simulink model "VSC_GFo_Fixed_Frequency_variable"  (R2016a)
settings: Solver=ode23tb  SolverMode=SingleTasking  StartTime=0.0  StopTime=2  FixedStep=Time_Step  MaxStep=1e-5  RelTol=1e-3
PreLoadFcn:
  | VSC_GFo_Init;
InitFcn:
  | VSC_GFo_Init;
values from neighbouring files (symbols this model uses):
  fb = fn    (= 50)    [VSC_GFo_Init.m]
  fn = 50    [VSC_GFo_Init.m]
  GRD00_Lg = GRD00_Xg/wb    (= 0.0254647908947)    [VSC_GFo_Init.m]
  GRD00_Rg = GRD00_Rg_pu*GRD00_Zb    (= 0.8)    [VSC_GFo_Init.m]
  Time_Step = 50e-6    (= 5e-05)    [VSC_GFo_Init.m]
  VSC01_Delta_P_Time_Step = 0.2    [VSC_GFo_Init.m]
  VSC01_Delta_P_Value = 0.2    [VSC_GFo_Init.m]
  VSC01_Udc_n = 640 * 1e3    (= 640000)    [VSC_GFo_Init.m]
undefined symbols (not defined in the file or in its folder): DiscIntNeverNeededParam, VSC01_id0
undefined symbols (not defined in the file): GRD00_H, GRD00_R, GRD00_TD, GRD00_TN, GRD00_Ub, VSC01_DX_DR, VSC01_I_thresh_pu, VSC01_Kp_Rvi_pu, VSC01_Lt_pu, VSC01_mp1, VSC01_mp2, VSC01_mp3, VSC01_Pn, VSC01_R, VSC01_Rt_pu, VSC01_Rv, VSC01_Sn, VSC01_T1, VSC01_T2, VSC01_Un1, VSC01_Un2, VSC01_W_LF, VSC01_wc1, VSC01_wc2, VSC01_wc3
libraries: powerlib x20, simulink x3, powerlib_meascontrol x1
(part 1 of 2)
settings Model: Creator=Frederic_Colas  LastModifiedBy=Frederic_Colas
settings DebuggingCC: UnconnectedInputMsg=none  UnconnectedOutputMsg=none  UnconnectedLineMsg=none  SFUnexpectedBacktrackingDiag=error  SFNoUnconditionalDefaultTransitionDiag=error
settings HardwareCC: ProdWordSize=32  ProdHWDeviceType=Specified
settings GRTTargetCC: TargetLangStandard=C99 (ISO)  GeneratePreprocessorConditionals=Use local settings
settings ConfigComp: CovMetricSettings=dwe  CovHtmlReporting=off  CovSaveCumulativeToWorkspaceVar=off  CovSaveSingleToWorkspaceVar=off  CovExternalEMLEnable=on
settings SimscapeCC: SimscapeNormalizeSystem=off

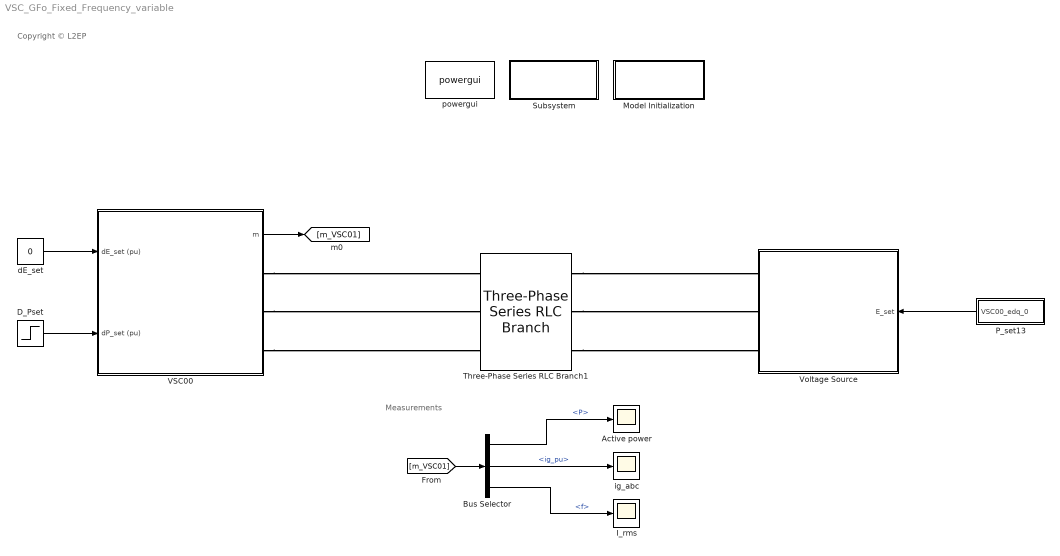
== system VSC_GFo_Fixed_Frequency_variable ==
  note: Copyright © L2EP
  note: Measurements
  Active power : Scope
  Bus Selector : BusSelector  OutputSignals=Control.P,ig_pu,Control.f
  D_Pset : Step  Time=VSC01_Delta_P_Time_Step  After=VSC01_Delta_P_Value  SampleTime=0
  I_rms : Scope
  Model Initialization : Subsystem  mask(Model Functions){InitFcnX=VSC_GFo_Init;, prel=on, posl=off, inif=on, strf=off}
      mask prompts: InitFcnX "Initialisation"; prel "Preload Function"; posl "PostLoad Function"; inif "InitFcn"; strf "StartFcn"
      mask init:
      | currentBlock = gcb;
      | root = bdroot(currentBlock);
      | 
      | if ~strcmp(get_param(root,'BlockDiagramType'),'library')
      |     if prel==1
      |         set_param(root, 'PreLoadFcn', InitFcnX);
      |     else
      |         set_param(root, 'PreLoadFcn', '');
      |     end
      |     if inif==1
      |         set_param(root, 'InitFcn', InitFcnX);
      |     else
      |         set_param(root, 'InitFcn', '');
      |     end
      |     if strf==1
      |         set_param(root, 'StartFcn', InitFcnX);
      |     else
      |         set_param(root, 'StartFcn', '');
      |     end
      |     if posl==1
      |         set_param(root, 'PostLoadFcn', InitFcnX);
      |     else
      |         set_param(root, 'PostLoadFcn', '');
      |     end
      | end
      | 
      | pos = get_param(currentBlock, 'Position');
      | width = pos(3) - pos(1); height = pos(4) - pos(2);
      | txt = [ upper(root) '\n' '- InitFcn. . . . . '  get_param(root, 'InitFcn') ];
      settings: CopyFcn=set_param(gcb,'LinkStatus','none')
      mask Display:
      | %text(5, height*0.5, txt, 'horizontalAlignment', 'left', 'verticalAlignment', 'middle') ;
      | color('blue'),disp('Initialization Function\nParameters')
  P_set13 : Subsystem
  Subsystem : Subsystem
      settings: OpenFcn=LoadFlow_VSC_v2
      mask Display: color('blue'),disp('Update Loadflow')
  Three-Phase Series RLC Branch1 : powerlib/Elements/Three-Phase Series RLC Branch  LConnTagsString=A|B|C  RConnTagsString=A|B|C  BranchType=RL  Resistance=GRD00_Rg  Inductance=GRD00_Lg  Capacitance=1e-6  Measurements=None
  VSC00 : Subsystem  mask(VSC){fb=fb, Sn=VSC01_Sn, Pn=VSC01_Pn, Vdcn=VSC01_Udc_n, Un1=VSC01_Un1, Un2=VSC01_Un2, Rt_pu=VSC01_Rt_pu, Lt_pu=VSC01_Lt_pu, Lm_pu=500, Rm_pu=500, Tr_PLL=100e-3, Val_Freq_Support=on, R_percent=VSC01_R, Rv=VSC01_Rv, W_TVR=VSC01_W_LF, I_thresh_pu=VSC01_I_thresh_pu, DX_DR=VSC01_DX_DR, Kp_Rvi_pu=VSC01_Kp_Rvi_pu, gainpopup=1, wc1=VSC01_wc1, mp1=VSC01_mp1, wc2=VSC01_wc2, mp2=VSC01_mp2, wc3=VSC01_wc3, mp3=VSC01_mp3, T1=VSC01_T1, T2=VSC01_T2, LFpopup=PQ, P0=0.5, Q0=5.2102e-06, V0=1, Theta0=1.4294}
      mask prompts: fb "Nominal Frequency (Hz)"; Sn "Nominal Apparent Power (VA)"; Pn "Nominal Power (W)"; Vdcn "Nominal DC Voltage (V)"; Un1 "VSC side Nominal Ph-Ph Voltage (V)"; Un2 "Grid side Nominal Ph-Ph Voltage (V)"; Rt_pu "R (pu)"; Lt_pu "L (pu)"; Lm_pu "Rm (pu)"; Rm_pu "Lm (pu)"; Tr_PLL "Time response (s)"; Val_Freq_Support "Frequency Support"; R_percent "Droop Gain (%)"; Rv "Damping Resistance (Rv)"; W_TVR "Dr filter"; I_thresh_pu "Current Threshold (pu)"; Kp_Rvi_pu "Kp_Rvi"; gainpopup "Strategy"; wc1 "wc"; mp1 "mp"; wc2 "wc"; mp2 "mp"; wc3 "wc"; mp3 "mp"; P0 "Initial Active Power (pu)"; Q0 "Initial Reactive Power (pu)"; V0 "Initial Voltage (pu)"; Theta0 "Initial Angle (°)"
      mask init:
      | % Update Name of LF bus for internal purpose
      |     NameStr = [get_param(gcb,'Name')];% '_LF'];
      |     set_param([gcb '/Load Flow Bus'],'ID',NameStr);
      |     %disp(NameStr);
      |     
      | % Increase size of Mask dialog box
      |    % pause(0.1);
      |     
      |     
      | % Base values
      |     %Un = Un1;
      |     Pb = Pn;
      |     cos_phi_n = Pn/Sn;
      |     Sb = Pb/cos_phi_n;
      |     %Ub = Un;
      |     Vn = Un1/sqrt(3);
      |     Vb = Vn;
      |     %Ib = Sb / Ub;
      |     Ib = Sb / (3*Vb);
      |     wb = 2*pi*fb;
      |   
      | % PLL derivation of the parameters
      |     wn_PLL=5/Tr_PLL;
      |     zeta_PLL = 1;
      |     Kp_PLL_pu = 2*zeta_PLL*wn_PLL/wb;
      |     Ki_PLL_pu = wn_PLL^2/wb;
      |     
      | % Set the chosen strategy
      |     Chosen_Strategy = gainpopup;
      |     
      | % Set the frequency droop gain
      |     R = R_percent;
      | 
      | % Compute Initial Voltage of VSC 
      | %   from steady-state output transformer model and Loadflow result
      |     if (LFpopup == 'PQ')
      |         V0 = 1;
      |     end
      |         
      |     R1_pu = Rt_pu/2;
      |     L1_pu = Lt_pu/2;
      |     R2_pu = Rt_pu/2;
      |     L2_pu = Lt_pu/2;
      |     X1_pu = L1_pu;
      |     X2_pu = L2_pu;
      |     Xm_pu = Lm_pu;
      |     
      |     Zm_pu = 1/(1/Rm_pu+1/(1i*Xm_pu));
      | 
      |     S0=P0+1i*Q0;
      |     I2 = conj(S0)/(V0);
      | 
      |     Vm = (R2_pu+1i*X2_pu)*I2 + V0;
      |     Im = Vm/Zm_pu;
      | 
      |     I1 = I2 + Im;
      |     V1 = (R1_pu+1i*X1_pu) * I1 + Vm;
      | 
      |     Vvsc0 = abs(V1);
      |    % disp(Vvsc0*1000)
      |     Theta_vsc0 = angle(V1) * 180/pi+Theta0;
      |     
      |     %vd0=Vvsc0*cos(Theta0*2*pi/180);
      |     %vq0=Vvsc0*sin(Theta0*2*pi/180); 
      |  
      |     %Va0 = Vvsc0*sqrt(2)*Ub/sqrt(3)*sin(Theta_vsc0*pi/180);
      |     %Vb0 = Vvsc0*sqrt(2)*Ub/sqrt(3)*sin(Theta_vsc0*pi/180-2*pi/3);
      |     %Vc0 = Vvsc0*sqrt(2)*Ub/sqrt(3)*sin(Theta_vsc0*pi/180+2*pi/3);
      |     
      |     Va0 = Vvsc0*sqrt(2)*Vb*sin(Theta_vsc0*pi/180);
      |     Vb0 = Vvsc0*sqrt(2)*Vb*sin(Theta_vsc0*pi/180-2*pi/3);
      |     Vc0 = Vvsc0*sqrt(2)*Vb*sin(Theta_vsc0*pi/180+2*pi/3);
      |     
      | % Generate string to display LF results on Mask
      |     %str_tmp = fprintf("Vvsc0 = %d, Theta_vsc0 = %d°",Vvsc0,Theta_vsc0);
      |     mo = get_param(gcb,'MaskObject');
      |     mo.getDialogControl('LF_vsc_str').Prompt = ['V0 = ', num2str(Vvsc0),' pu, Angle = ', num2str(Theta_vsc0),'°'];
      |     mo.getDialogControl('LF_pcc_str').Prompt = ['V0 = ', num2str(V0),' pu, Angle = ', num2str(Theta0),'°'];
      |     mo.getDialogControl('LF_pcc_Power_str').Prompt = ['P0 = ', num2str(P0),' pu, Q0 = ', num2str(Q0),' pu'];
      |     %set_param([gcb],'LF_str',str_tmp);
      |  %GRD00_Theta0 = Theta0;
      |  %P0 = 200e6;
      |  %Q0 = 0;
      |  % Initial current values of VSC (dq pu) 
      |  %id0 =(P0*vd0+Q0*vq0)/(vd0^2+vq0^2) * 1/Ib; %
      |  %iq0 =(P0*vq0-Q0*vd0)/(vd0^2+vq0^2) * 1/Ib; %Initial current in the connexion inductance
      settings: OpenFcn=|
      | NameStr = get_param(gcb,'Name');
      | open_system(gcbh, 'Mask');
      | 
      | h2AllOpenDlgs = DAStudio.ToolRoot.getOpenDialogs;
      | 
      | for i=1:length(h2AllOpenDlgs)
      |     try
      |          %disp(h2AllOpenDlgs(i).getSource.getBlock.Name);
      |         Dialog_block_name = h2AllOpenDlgs(i).getSource.getBlock.Name;
      |          %strcmp(Dialog_block_name, NameStr),
      |         if (strcmp(h2AllOpenDlgs(i).getSource.getBlock.Name, NameStr))
      |             iPos = h2AllOpenDlgs(i).position;
      |             h2AllOpenDlgs(i).position = [iPos(1)   iPos(2)   iPos(3)*1.4   iPos(4)];
      |         end
      |     end
      | end
      mask TypeOptions gainpopup: 1 | 2 | 3
      mask Callback gainpopup:
      | % Get the mask parameter values. This is a cell
      | %   array of character vectors.
      | maskStr = get_param(gcb,'gainpopup');
      | p=Simulink.Mask.get(gcb);
      | 
      | % The pop-up menu is the first mask parameter.
      | %   Check the value selected in the pop-up
      | if strcmp(maskStr,'1'),
      | 
      |     % Set the visibility of both parameters on when
      |     %   User-defined is selected in the pop-up.
      |     p.getDialogControl('Param_Strat_1').Visible='on';
      |     p.getDialogControl('Param_Strat_2').Visible='off';
      |     p.getDialogControl('Param_Strat_3').Visible='off';
      | 
      | elseif strcmp(maskStr,'2'),
      | 
      |     % Set the visibility of both parameters on when
      |     %   User-defined is selected in the pop-up.
      |     p.getDialogControl('Param_Strat_1').Visible='off';
      |     p.getDialogControl('Param_Strat_2').Visible='on';
      |     p.getDialogControl('Param_Strat_3').Visible='off';
      | 
      |     % Turn off the visibility of the Value field
      |     %   when User-defined is not selected.
      | else
      | 
      |     % Set the visibility of both parameters on when
      |     %   User-defined is selected in the pop-up.
      |     p.getDialogControl('Param_Strat_1').Visible='off';
      |     p.getDialogControl('Param_Strat_2').Visible='off';
      |     p.getDialogControl('Param_Strat_3').Visible='on';
      | 
      | end
      mask TypeOptions LFpopup: Swing | PQ | PV
      mask Callback LFpopup:
      | % Get the mask parameter values. This is a cell
      | %   array of character vectors.
      | maskStr = get_param(gcb,'LFpopup');
      | p=Simulink.Mask.get(gcb);
      | 
      | % The pop-up menu is the first mask parameter.
      | %   Check the value selected in the pop-up
      | if strcmp(maskStr,'Swing'),
      | 
      |     % Set the visibility of both parameters on when
      |     %   User-defined is selected in the pop-up.
      |     p.getParameter('P0').Visible='off';
      |     p.getParameter('Q0').Visible='off';
      |     p.getParameter('V0').Visible='on';
      |     p.getParameter('Theta0').Visible='on';
      |     set_param([gcb '/Source_For_LF'],'BusType','swing');
      | 
      | elseif strcmp(maskStr,'PQ'),
      | 
      |     % Set the visibility of both parameters on when
      |     %   User-defined is selected in the pop-up.
      |     p.getParameter('P0').Visible='on';
      |     p.getParameter('Q0').Visible='on';
      |     p.getParameter('V0').Value='1';
      |     set_param(gcb,'V0','1');
      |     p.getParameter('V0').Visible='off';
      |     p.getParameter('Theta0').Visible='off';
      |     set_param([gcb '/Source_For_LF'],'BusType','PQ');
      | 
      |     % Turn off the visibility of the Value field
      |     %   when User-defined is not selected.
      | else
      | 
      |     % Set the visibility of both parameters on when
      |     %   User-defined is selected in the pop-up.
      |     p.getParameter('P0').Visible='on';
      |     p.getParameter('Q0').Visible='off';
      |     p.getParameter('V0').Visible='on';
      |     p.getParameter('Theta0').Visible='off';
      |     set_param([gcb '/Source_For_LF'],'BusType','PV');
      | 
      | end
      mask DialogControl Title_Strat_1 Prompt: Strategy 1
      mask DialogControl Title_Strat_2 Prompt: Strategy 2
      mask DialogControl Title_Strat_3 Prompt: Strategy 3
      mask DialogControl Control4 Prompt: Initial Operating Point
      mask DialogControl Container24 Prompt: VSC side
      mask DialogControl LF_vsc_str Prompt: V0 = 1.0055 pu, Angle = 5.7158°
      mask DialogControl Container25 Prompt: PCC
      mask DialogControl UpdateLoadflow Prompt: Update Loadflow
      mask DialogControl UpdateLoadflow Callback: Load_Flow_VSC
      mask Display:
      | disp('L-Filter');
      | port_label('input',1,'dE_set (pu)');
      | port_label('input',2,'dP_set (pu)');
      | port_label('output',1,'m');
      | port_label('rconn',1,'A');
      | port_label('rconn',2,'B');
      | port_label('rconn',3,'C');
  Voltage Source : Subsystem  mask(Inertial_Voltage_source){fb=fb, Sc=1e9, Ub=GRD00_Ub, H_eq=GRD00_H, Droop=GRD00_R, TN=GRD00_TN, TD=GRD00_TD}
      mask prompts: fb "Nominal Frequency (Hz)"; Sc "Nominal Power (VA)"; Ub "Nominal Voltage (V)"; H_eq "Inertial Constant H (s)"; Droop "Droop Gain"; TN "Lead Time Constant"; TD "Lag Time Constant"
      mask init:
      | % Base values
      |     wb=2*pi*fb;
      |     Ib=Sc/(sqrt(3)*Ub);
      |     Vb=Ub/sqrt(3);
      |     e0=Vb;
      |     Theta_e0=0;
      |   
      | % Parameters
      |     R=Droop;
      mask DialogControl Container5 Prompt: Nominal Values
      mask DialogControl Container16 Prompt: Network Time Constants
  dE_set : Constant  Value=0
  ig_abc : Scope
  powergui : powerlib/powergui  Priority=1  SimulationMode=Discrete  SampleTime=Time_Step/2  frequency=60  Iterations=50  frequencyindice=50  Pbase=1000e6  ErrMax=1e-4  UnitsV=kV  UnitsW=MW  buscounter=0  FunctionMessages=off  echomessages=off  EnableUseOfTLC=off  CurrentSourceSwitches=off  DisableSnubberDevices=off  DisableRonSwitches=off  DisableVfSwitches=off  DisplayEquations=off  SolverType=Tustin/Backward Euler (TBE)  Interpol=off  ExternalGateDelay=off  methode=off  Ts=100  x0status=blocks  SPID=on  SwTol=0  HookPort=off  RestoreLinks=warning  ResistiveCurrentMeasurement=off  Frange=[0:2:500]  Ylog=off  Xlog=on  ShowGrid=off  save=off  variable=ZData  structure=0  ZoomFFT=off  StartTime=0.0  cycles=1  DisplayStyle=1  fundamental=60  FreqAxis=off  MaxFrequency=1000  frequencyindicesteady=1  RmsSteady=1  display=off
  wires:
  dE_set/1 -> VSC00/1(dE_set (pu))
  D_Pset/1 -> VSC00/2(dP_set (pu))
  [m_VSC01] -> Bus Selector/1
  P_set13/1(VSC00_edq_0) -> Voltage Source/1(E_set)
  Bus Selector/1 -> Active power/1  "<P>"
  VSC00/1(m) -> [m_VSC01]
  Bus Selector/2 -> ig_abc/1  "<ig_pu>"
  Bus Selector/3 -> I_rms/1  "<f>"
  connections:
  VSC00/RConn1 -- Three-Phase Series RLC Branch1/LConn1
  VSC00/RConn3 -- Three-Phase Series RLC Branch1/LConn3
  VSC00/RConn2 -- Three-Phase Series RLC Branch1/LConn2
  Three-Phase Series RLC Branch1/RConn2 -- Voltage Source/RConn2
  Three-Phase Series RLC Branch1/RConn1 -- Voltage Source/RConn1
  Three-Phase Series RLC Branch1/RConn3 -- Voltage Source/RConn3

== system VSC_GFo_Fixed_Frequency_variable/Model Initialization ==

== system VSC_GFo_Fixed_Frequency_variable/P_set13 ==
  Mux : Mux  Inputs=2
  ed1 : Constant  Value=0
  eq1 : Constant
  VSC00_edq_0 : Outport
  wires:
  Mux/1 -> VSC00_edq_0/1
  eq1/1 -> Mux/1
  ed1/1 -> Mux/2

== system VSC_GFo_Fixed_Frequency_variable/Subsystem ==

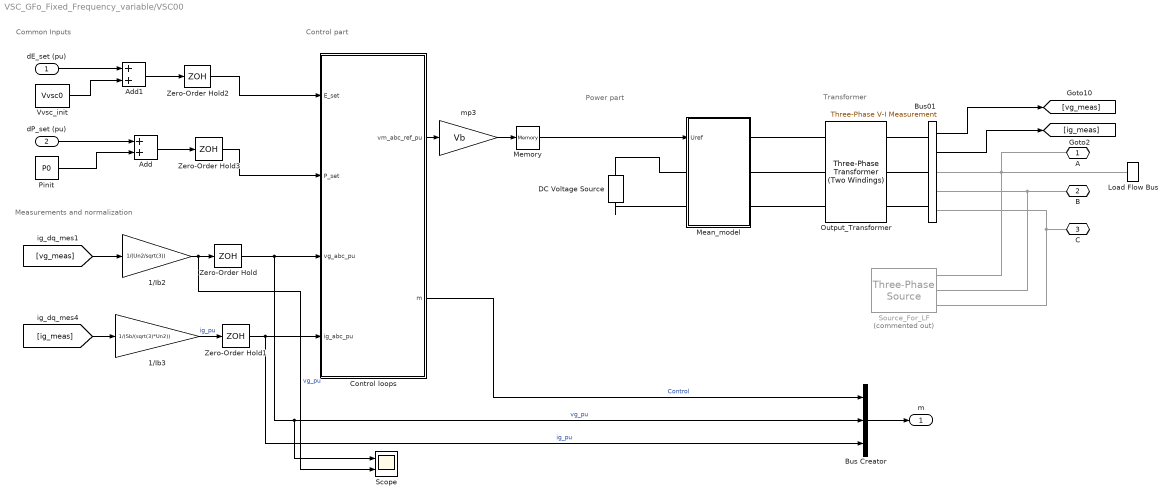
== system VSC_GFo_Fixed_Frequency_variable/VSC00 ==
  note: Transformer
  note: Common Inputs
  note: Power part
  note: Measurements and normalization
  note: Control part
  dE_set (pu) : Inport
  dP_set (pu) : Inport  Port=2
  1/Ib2 : Gain  Gain=1/(Un2/sqrt(3))
  1/Ib3 : Gain  Gain=1/(Sb/(sqrt(3)*Un2))
  Add : Sum
  Add1 : Sum
  Bus Creator : BusCreator  Inputs=3
  Bus01 : powerlib/Measurements/Three-Phase V-I Measurement  VoltageMeasurement=phase-to-ground  SetLabelV=off  LabelV=Vabc  Vpu=off  VpuLL=off  CurrentMeasurement=yes  SetLabelI=off  LabelI=Iabc  Ipu=off  Pbase=100e6  Vbase=500e3  OutputType=Complex  PhasorSimulation=off  PSBequivalent=0
  Control loops : Subsystem
  DC Voltage Source : powerlib/Electrical Sources/DC Voltage Source  Amplitude=VSC01_Udc_n  Measurements=Voltage
  Load Flow Bus : powerlib/Measurements/Load Flow Bus  LConnTagsString=a  Phases=single  Connectors=on one side  ID=VSC00  Vbase=Un2  Vref=V0  Vangle=Theta0  VLF=1.002  VLFb=1  VLFc=1  angleLF=1.429  angleLFb=0  angleLFc=0
  Mean_model : Subsystem
  Memory : Memory  X0=[Va0 Vb0 Vc0]  InheritSampleTime=on
  Output_Transformer : powerlib/Elements/Three-Phase Transformer (Two Windings)  Winding1Connection=Yg  Winding2Connection=Yg  CoreType=Three single-phase transformers  SetSaturation=off  Hysteresis=off  DataFile='hysteresis'  SetInitialFlux=off  Measurements=None  UNITS=pu  NominalPower=[Sn , fn ]  Winding1=[Un1 , Rt_pu/2 , Lt_pu/2]  Winding2=[Un2 , Rt_pu/2 , Lt_pu/2]  Rm=Rm_pu  Lm=Lm_pu  L0=0.5  Saturation=[ 0,0 ; 0.0024,1.2 ; 1.0,1.52 ]  InitialFluxes=[ 0.8 , -0.8 , 0.7 ]  MoreParameters=off  BreakLoop=off  DataType=off  TransfoNumber=1
  Pinit : Constant  Value=P0
  Scope : Scope  NumInputPorts=2
  Source_For_LF : powerlib/Electrical Sources/Three-Phase Source  Commented=on  InternalConnection=Yg  VoltagePhases=off  Voltage=(400000)*1.00218  PhaseAngle=1.4294  Voltage_phases=[25e3 25e3 25e3]/sqrt(3)  PhaseAngles_phases=[0 -120 +120]  Frequency=fb  NonIdealSource=off  SpecifyImpedance=off  Resistance=0  Inductance=0  ShortCircuitLevel=100e6  BaseVoltage=Un  XRratio=7  BusType=PQ  Pref=P0*Sb  Qref=Q0*Sb  Prefabc=[10e3, 10e3, 10e3]  Qrefabc=[0, 0, 0]  Qmin=-inf  Qmax=inf
  Vvsc_init : Constant  Value=Vvsc0
  Zero-Order Hold{,1..3} (4 alike) : ZeroOrderHold  SampleTime=Time_Step
  mp3 : Gain  Gain=Vb
  A : PMIOPort  Port=1  Side=Right
  B : PMIOPort  Port=2  Side=Right
  C : PMIOPort  Port=3  Side=Right
  m : Outport
  wires:
  Add/1 -> Zero-Order Hold3/1
  Control loops/2(m) -> Bus Creator/1  "Control"
  1/Ib3/1 -> Zero-Order Hold1/1  "ig_pu"
  1/Ib2/1 -> Scope/2, Zero-Order Hold/1  "vg_pu"
  Bus Creator/1 -> m/1
  [vg_meas] -> 1/Ib2/1
  Control loops/1(vm_abc_ref_pu) -> mp3/1
  Add1/1 -> Zero-Order Hold2/1
  dP_set (pu)/1 -> Add/1
  Pinit/1 -> Add/2
  Vvsc_init/1 -> Add1/2
  Bus01/1 -> [vg_meas]
  dE_set (pu)/1 -> Add1/1
  Bus01/2 -> [ig_meas]
  [ig_meas] -> 1/Ib3/1
  Zero-Order Hold/1 -> Scope/1, Bus Creator/2, Control loops/3(vg_abc_pu)  "vg_pu"
  Zero-Order Hold1/1 -> Bus Creator/3, Control loops/4(ig_abc_pu)  "ig_pu"
  Zero-Order Hold2/1 -> Control loops/1(E_set)
  Zero-Order Hold3/1 -> Control loops/2(P_set)
  mp3/1 -> Memory/1
  Memory/1 -> Mean_model/1(Uref)
  connections:
  DC Voltage Source/LConn1 -- Mean_model/LConn2
  Output_Transformer/RConn1 -- Bus01/LConn1
  Output_Transformer/RConn2 -- Bus01/LConn2
  DC Voltage Source/RConn1 -- Mean_model/LConn1
  Output_Transformer/RConn3 -- Bus01/LConn3
  Source_For_LF/RConn2 -- B/RConn1 -- Bus01/RConn2
  Mean_model/RConn1 -- Output_Transformer/LConn1
  Mean_model/RConn2 -- Output_Transformer/LConn2
  Mean_model/RConn3 -- Output_Transformer/LConn3
  Source_For_LF/RConn1 -- Load Flow Bus/LConn1 -- A/RConn1 -- Bus01/RConn1
  Source_For_LF/RConn3 -- C/RConn1 -- Bus01/RConn3

== system VSC_GFo_Fixed_Frequency_variable/Voltage Source ==
  E_set : Inport
  Load Flow Bus : powerlib/Measurements/Load Flow Bus  LConnTagsString=a  Phases=single  Connectors=on one side  ID=BUS_1  Vbase=Ub  Vref=1  Vangle=0  VLF=1  VLFb=1  VLFc=1  angleLF=0  angleLFb=0  angleLFc=0
  Mean_model : Subsystem
  Source_For_LF : powerlib/Electrical Sources/Three-Phase Source  Commented=on  InternalConnection=Yg  VoltagePhases=off  Voltage=(400000)*1  PhaseAngle=0  Voltage_phases=[25e3 25e3 25e3]/sqrt(3)  PhaseAngles_phases=[0 -120 +120]  Frequency=fb  NonIdealSource=on  SpecifyImpedance=off  Resistance=0  Inductance=0  ShortCircuitLevel=100e6  BaseVoltage=GRD00_Un  XRratio=7  BusType=swing  Pref=P0  Qref=Q0  Prefabc=[10e3, 10e3, 10e3]  Qrefabc=[0, 0, 0]  Qmin=-inf  Qmax=inf
  Voltage generation : Subsystem
  A : PMIOPort  Port=1  Side=Right
  B : PMIOPort  Port=2  Side=Right
  C : PMIOPort  Port=3  Side=Right
  wires:
  E_set/1 -> Voltage generation/1(E_set)
  Voltage generation/1(vg_abc) -> Mean_model/1(u_abc)
  connections:
  Mean_model/RConn3 -- C/RConn1 -- Source_For_LF/RConn3
  Mean_model/RConn2 -- B/RConn1 -- Source_For_LF/RConn2
  Mean_model/RConn1 -- A/RConn1 -- Source_For_LF/RConn1 -- Load Flow Bus/LConn1

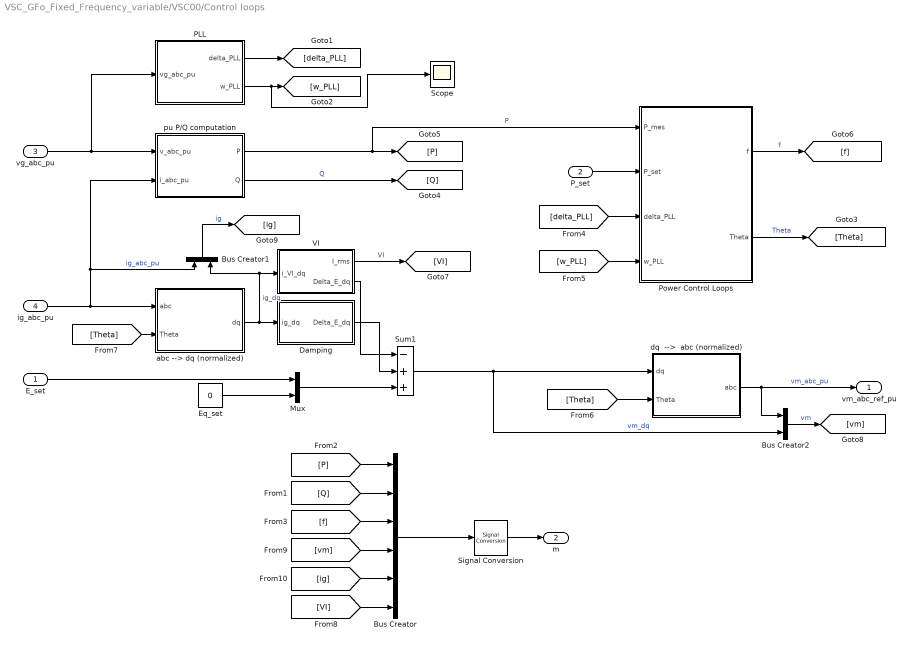
== system VSC_GFo_Fixed_Frequency_variable/VSC00/Control loops ==
  E_set : Inport
  P_set : Inport  Port=2
  vg_abc_pu : Inport  Port=3
  ig_abc_pu : Inport  Port=4
  " pu P/Q computation" : Subsystem  DialogController=POWERSYS.PowerSysDialog
  Bus Creator : BusCreator  Inputs=6
  Bus Creator1 : BusCreator  Inputs=2
  Bus Creator2 : BusCreator  Inputs=2
  Damping : Subsystem
  Eq_set : Constant  Value=0
  Mux : Mux  Inputs=2
  PLL : Subsystem
  Power Control Loops : Subsystem
  Scope : Scope
  Signal Conversion : SignalConversion  OverrideOpt=off
  Sum1 : Sum  Inputs=-++
  VI : Subsystem
  abc --> dq (normalized) : Subsystem
  "dq  -->  abc (normalized) " : Subsystem
  vm_abc_ref_pu : Outport
  m : Outport  Port=2
  wires:
  [ig] -> Bus Creator/5
  Bus Creator1/1 -> [ig]  "ig"
  Bus Creator/1 -> Signal Conversion/1
  [VI] -> Bus Creator/6
  [vm] -> Bus Creator/4
  Bus Creator2/1 -> [vm]  "vm"
  Eq_set/1 -> Mux/2
  Mux/1 -> Sum1/3
  VI/1(I_rms) -> [VI]  "VI"
  Damping/1("Delta_E_dq ") -> Sum1/2
  VI/2(Delta_E_dq) -> Sum1/1
  [Theta] -> abc --> dq (normalized)/2(Theta)
  [Theta] -> "dq  -->  abc (normalized) "/2(Theta)
  Power Control Loops/2(Theta) -> [Theta]  "Theta"
  abc --> dq (normalized)/1(dq) -> Bus Creator1/2, VI/1(i_VI_dq), Damping/1(ig_dq)  "ig_dq"
  ig_abc_pu/1 -> abc --> dq (normalized)/1(abc), " pu P/Q computation"/2(i_abc_pu), Bus Creator1/1  "ig_abc_pu"
  " pu P/Q computation"/1(P) -> [P], Power Control Loops/1(P_mes)  "P"
  PLL/2(w_PLL) -> Scope/1, [w_PLL]
  PLL/1(delta_PLL) -> [delta_PLL]
  vg_abc_pu/1 -> " pu P/Q computation"/1(v_abc_pu), PLL/1(vg_abc_pu)
  Power Control Loops/1(f) -> [f]  "f"
  [w_PLL] -> Power Control Loops/4(w_PLL)
  P_set/1 -> Power Control Loops/2(P_set)
  [delta_PLL] -> Power Control Loops/3(delta_PLL)
  Sum1/1 -> "dq  -->  abc (normalized) "/1(dq), Bus Creator2/2  "vm_dq"
  " pu P/Q computation"/2(Q) -> [Q]  "Q"
  E_set/1 -> Mux/1
  "dq  -->  abc (normalized) "/1(abc) -> Bus Creator2/1, vm_abc_ref_pu/1  "vm_abc_pu"
  [f] -> Bus Creator/3
  [Q] -> Bus Creator/2
  [P] -> Bus Creator/1
  Signal Conversion/1 -> m/1

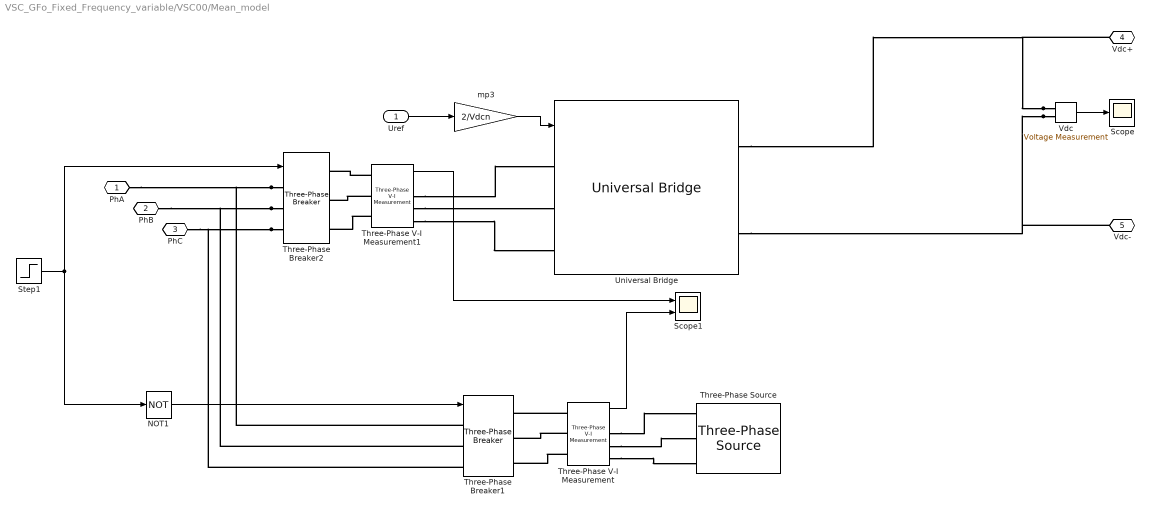
== system VSC_GFo_Fixed_Frequency_variable/VSC00/Mean_model ==
  Uref : Inport
  NOT1 : Logic  Operator=NOT  IconShape=distinctive  AllPortsSameDT=off  OutDataTypeStr=boolean
  Scope : Scope
  Scope1 : Scope  NumInputPorts=2
  Step1 : Step  Time=Time_Step  SampleTime=Time_Step
  Three-Phase V-I Measurement : powerlib/Measurements/Three-Phase V-I Measurement  VoltageMeasurement=phase-to-ground  SetLabelV=off  LabelV=Vabc  Vpu=off  VpuLL=off  CurrentMeasurement=yes  SetLabelI=off  LabelI=Iabc  Ipu=off  Pbase=100e6  Vbase=500e3  OutputType=Complex  PhasorSimulation=off  PSBequivalent=0
  Three-Phase V-I Measurement1 : powerlib/Measurements/Three-Phase V-I Measurement  VoltageMeasurement=phase-to-ground  SetLabelV=off  LabelV=Vabc  Vpu=off  VpuLL=off  CurrentMeasurement=yes  SetLabelI=off  LabelI=Iabc  Ipu=off  Pbase=100e6  Vbase=500e3  OutputType=Complex  PhasorSimulation=off  PSBequivalent=0
  Three-Phase Breaker1 : powerlib/Elements/Three-Phase Breaker  InitialState=closed  SwitchA=on  SwitchB=on  SwitchC=on  SwitchTimes="[4/60  10/60]"  External=on  BreakerResistance=0.001  SnubberResistance=1e6  SnubberCapacitance=inf  Measurements=None
  Three-Phase Breaker2 : powerlib/Elements/Three-Phase Breaker  InitialState=open  SwitchA=on  SwitchB=on  SwitchC=on  SwitchTimes="[4/60  10/60]"  External=on  BreakerResistance=0.001  SnubberResistance=1e6  SnubberCapacitance=inf  Measurements=None
  Three-Phase Source : powerlib/Electrical Sources/Three-Phase Source  InternalConnection=Yg  VoltagePhases=off  Voltage=Vvsc0*Un1  PhaseAngle=Theta_vsc0  Voltage_phases=[25e3 25e3 25e3]/sqrt(3)  PhaseAngles_phases=[0 -120 +120]  Frequency=fb  NonIdealSource=off  SpecifyImpedance=off  Resistance=0  Inductance=0  ShortCircuitLevel=100e6  BaseVoltage=VSC01_Un1  XRratio=7  BusType=swing  Pref=0.3  Qref=0  Prefabc=[10e3, 10e3, 10e3]  Qrefabc=[0, 0, 0]  Qmin=-Inf  Qmax=Inf
  Universal Bridge : powerlib/Power Electronics/Universal Bridge  Arms=3  SnubberResistance=1e5  SnubberCapacitance=inf  Device=Average-model based VSC  Ron=1e-3  Lon=0  ForwardVoltages="[  0  0  ]"  ForwardVoltage=0  GTOparameters=[ 10e-6 , 20e-6 ]  IGBTparameters=[ 1e-6 , 2e-6 ]  Measurements=None  Measurements_2=None  converterType=Rectifier
  Vdc : powerlib/Measurements/Voltage Measurement  PhasorSimulation=off  OutputType=Complex  PSBequivalent=0
  mp3 : Gain  Gain=2/Vdcn
  PhA : PMIOPort  Port=1  Side=Right
  PhB : PMIOPort  Port=2  Side=Right
  PhC : PMIOPort  Port=3  Side=Right
  Vdc+ : PMIOPort  Port=4  Side=Left
  Vdc- : PMIOPort  Port=5  Side=Left
  wires:
  NOT1/1 -> Three-Phase Breaker1/1
  Step1/1 -> NOT1/1, Three-Phase Breaker2/1
  mp3/1 -> Universal Bridge/1
  Uref/1 -> mp3/1
  Vdc/1 -> Scope/1
  Three-Phase V-I Measurement1/1 -> Scope1/1
  Three-Phase V-I Measurement/1 -> Scope1/2
  connections:
  Three-Phase Breaker2/LConn1 -- Three-Phase Breaker1/LConn1 -- PhA/RConn1
  Three-Phase Breaker2/LConn2 -- Three-Phase Breaker1/LConn2 -- PhB/RConn1
  Three-Phase Breaker2/LConn3 -- Three-Phase Breaker1/LConn3 -- PhC/RConn1
  Vdc/LConn1 -- Universal Bridge/RConn1 -- Vdc+/RConn1
  Vdc/LConn2 -- Universal Bridge/RConn2 -- Vdc-/RConn1
  Three-Phase V-I Measurement/LConn1 -- Three-Phase Breaker1/RConn1
  Three-Phase V-I Measurement/LConn2 -- Three-Phase Breaker1/RConn2
  Three-Phase V-I Measurement/LConn3 -- Three-Phase Breaker1/RConn3
  Three-Phase V-I Measurement/RConn3 -- Three-Phase Source/RConn3
  Three-Phase V-I Measurement/RConn2 -- Three-Phase Source/RConn2
  Three-Phase V-I Measurement/RConn1 -- Three-Phase Source/RConn1
  Three-Phase V-I Measurement1/LConn1 -- Three-Phase Breaker2/RConn1
  Three-Phase V-I Measurement1/LConn2 -- Three-Phase Breaker2/RConn2
  Three-Phase V-I Measurement1/LConn3 -- Three-Phase Breaker2/RConn3
  Three-Phase V-I Measurement1/RConn2 -- Universal Bridge/LConn2
  Three-Phase V-I Measurement1/RConn3 -- Universal Bridge/LConn3
  Three-Phase V-I Measurement1/RConn1 -- Universal Bridge/LConn1

== system VSC_GFo_Fixed_Frequency_variable/Voltage Source/Mean_model ==
  u_abc : Inport
  Controlled Voltage Source1 : powerlib/Electrical Sources/Controlled Voltage Source  Initialize=on  Source_Type=AC  Amplitude=e0*sqrt(2)  Phase=0  Frequency=fb  Measurements=None
  Controlled Voltage Source2 : powerlib/Electrical Sources/Controlled Voltage Source  Initialize=on  Source_Type=AC  Amplitude=e0*sqrt(2)  Phase=-240  Frequency=fb  Measurements=None
  Controlled Voltage Source4 : powerlib/Electrical Sources/Controlled Voltage Source  Initialize=on  Source_Type=AC  Amplitude=e0*sqrt(2)  Phase=-120  Frequency=fb  Measurements=None
  Demux : Demux  Outputs=3
  Ground2 : powerlib/Elements/Ground  LConnTagsString=a
  A : PMIOPort  Port=1  Side=Right
  B : PMIOPort  Port=2  Side=Right
  C : PMIOPort  Port=3  Side=Right
  wires:
  u_abc/1 -> Demux/1
  Demux/2 -> Controlled Voltage Source4/1
  Demux/3 -> Controlled Voltage Source2/1
  Demux/1 -> Controlled Voltage Source1/1
  connections:
  Controlled Voltage Source4/LConn1 -- Controlled Voltage Source1/LConn1 -- Controlled Voltage Source2/LConn1 -- Ground2/LConn1
  Controlled Voltage Source2/RConn1 -- C/RConn1
  Controlled Voltage Source4/RConn1 -- B/RConn1
  Controlled Voltage Source1/RConn1 -- A/RConn1

== system VSC_GFo_Fixed_Frequency_variable/Voltage Source/Voltage generation ==
  E_set : Inport
  Mux : Mux  Inputs=3
  Voltage generation : Subsystem
  pu --> SI : Subsystem
  vg_abc : Outport
  wires:
  pu --> SI/1(e_a_SI) -> Mux/1
  Voltage generation/3(v_c) -> pu --> SI/3(e_c_pu)
  Mux/1 -> vg_abc/1
  pu --> SI/3(e_c_SI) -> Mux/3
  pu --> SI/2(e_b_SI) -> Mux/2
  Voltage generation/1(v_a) -> pu --> SI/1(e_a_pu)
  Voltage generation/2(v_b) -> pu --> SI/2(e_b_pu)
  E_set/1 -> Voltage generation/1(E_set)

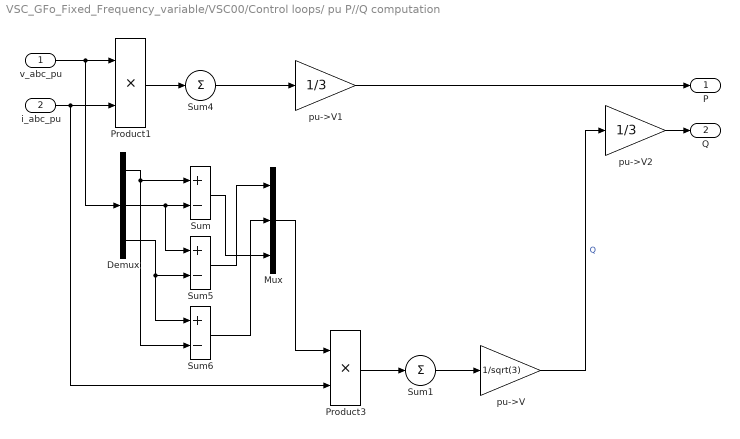
== system VSC_GFo_Fixed_Frequency_variable/VSC00/Control loops/ pu P//Q computation ==
  v_abc_pu : Inport  PortDimensions=3
  i_abc_pu : Inport  Port=2  PortDimensions=3
  Demux : Demux  Outputs=3
  Mux : Mux  Inputs=3
  Product1 : Product  SaturateOnIntegerOverflow=on  InputSameDT=on  OutDataTypeStr=Inherit: Same as first input
  Product3 : Product  SaturateOnIntegerOverflow=on  InputSameDT=on  OutDataTypeStr=Inherit: Same as first input
  Sum : Sum  Inputs=+-  SaturateOnIntegerOverflow=on  InputSameDT=on  OutDataTypeStr=Inherit: Same as first input
  Sum1 : Sum  Inputs=1  SaturateOnIntegerOverflow=on  InputSameDT=on  OutDataTypeStr=Inherit: Same as first input
  Sum4 : Sum  Inputs=1  SaturateOnIntegerOverflow=on  InputSameDT=on  OutDataTypeStr=Inherit: Same as first input
  Sum5 : Sum  Inputs=+-  SaturateOnIntegerOverflow=on  InputSameDT=on  OutDataTypeStr=Inherit: Same as first input
  Sum6 : Sum  Inputs=+-  SaturateOnIntegerOverflow=on  InputSameDT=on  OutDataTypeStr=Inherit: Same as first input
  pu->V : Gain  Gain=1/sqrt(3)  SaturateOnIntegerOverflow=on  OutDataTypeStr=Inherit: Same as input  ParamDataTypeStr=Inherit: Same as input
  pu->V1 : Gain  Gain=1/3  SaturateOnIntegerOverflow=on  OutDataTypeStr=Inherit: Same as input  ParamDataTypeStr=Inherit: Same as input
  pu->V2 : Gain  Gain=1/3  SaturateOnIntegerOverflow=on  OutDataTypeStr=Inherit: Same as input  ParamDataTypeStr=Inherit: Same as input
  P : Outport
  Q : Outport  Port=2
  wires:
  pu->V2/1 -> Q/1
  pu->V1/1 -> P/1
  Sum1/1 -> pu->V/1
  Product3/1 -> Sum1/1
  Product1/1 -> Sum4/1
  v_abc_pu/1 -> Product1/1, Demux/1
  i_abc_pu/1 -> Product1/2, Product3/2
  Sum4/1 -> pu->V1/1
  Demux/1 -> Sum/1, Sum6/2
  Demux/2 -> Sum/2, Sum5/1
  Demux/3 -> Sum5/2, Sum6/1
  Sum/1 -> Mux/3
  Sum5/1 -> Mux/1
  Sum6/1 -> Mux/2
  Mux/1 -> Product3/1
  pu->V/1 -> pu->V2/1  "Q"

== system VSC_GFo_Fixed_Frequency_variable/VSC00/Control loops/Damping ==
  ig_dq : Inport
  Filter w_LF : Subsystem
      mask Display: disp('\omega_{LF} / (s + \omega_{LF})','texmode','on')
  Sum5 : Sum  Inputs=|+-
  Zero-Order Hold : ZeroOrderHold  SampleTime=Time_Step
  nq1 : Gain  Gain=Rv
  "Delta_E_dq " : Outport
  wires:
  nq1/1 -> Filter w_LF/1(e), Sum5/2
  Filter w_LF/1(s) -> Sum5/1
  Sum5/1 -> Zero-Order Hold/1
  ig_dq/1 -> nq1/1
  Zero-Order Hold/1 -> "Delta_E_dq "/1

== system VSC_GFo_Fixed_Frequency_variable/VSC00/Control loops/PLL ==
  vg_abc_pu : Inport
  Demux : Demux  Outputs=2
  PI PLL controller : Subsystem
  Terminator : Terminator
  abc --> dq (normalized) : Subsystem
  delta_PLL : Outport
  w_PLL : Outport  Port=2
  wires:
  abc --> dq (normalized)/1(dq) -> Demux/1
  vg_abc_pu/1 -> abc --> dq (normalized)/1(abc)
  PI PLL controller/2(delta_theta) -> delta_PLL/1, abc --> dq (normalized)/2(Theta)
  Demux/1 -> Terminator/1
  PI PLL controller/1(w_PLL) -> w_PLL/1
  Demux/2 -> PI PLL controller/1(Vq)

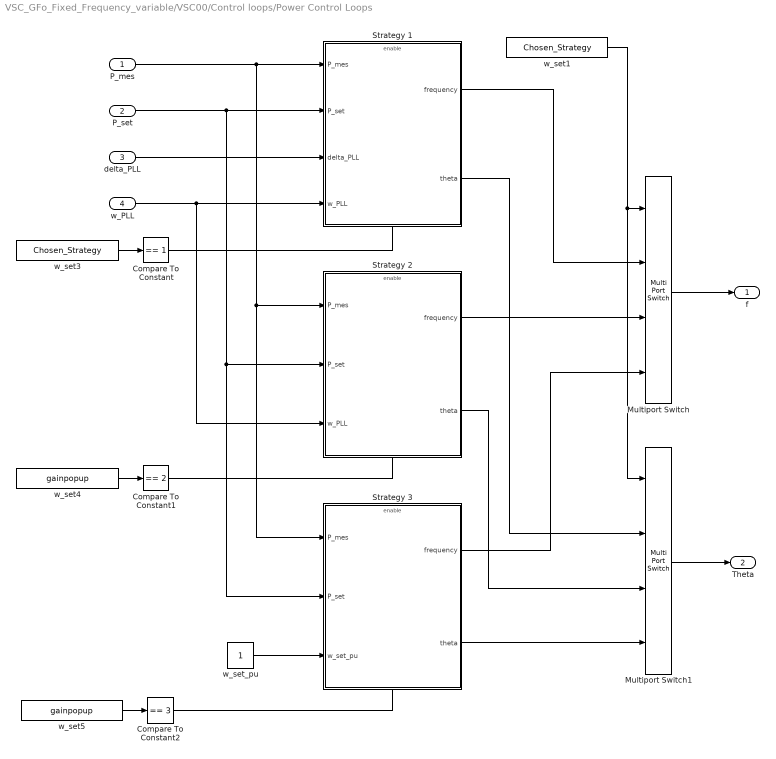
== system VSC_GFo_Fixed_Frequency_variable/VSC00/Control loops/Power Control Loops ==
  P_mes : Inport
  P_set : Inport  Port=2
  delta_PLL : Inport  Port=3
  w_PLL : Inport  Port=4
  Compare To Constant : simulink/Logic and Bit Operations/Compare To Constant  relop===  const=1  OutDataTypeStr=boolean
  Compare To Constant1 : simulink/Logic and Bit Operations/Compare To Constant  relop===  const=2  OutDataTypeStr=boolean
  Compare To Constant2 : simulink/Logic and Bit Operations/Compare To Constant  relop===  const=3  OutDataTypeStr=boolean
  Multiport Switch : MultiPortSwitch
  Multiport Switch1 : MultiPortSwitch
  Strategy 1 : Subsystem
  Strategy 2 : Subsystem
  Strategy 3 : Subsystem
  w_set1 : Constant  Value=Chosen_Strategy
  w_set3 : Constant  Value=Chosen_Strategy
  w_set4 : Constant  Value=gainpopup
  w_set5 : Constant  Value=gainpopup
  w_set_pu : Constant
  f : Outport
  Theta : Outport  Port=2
  wires:
  Compare To Constant2/1 -> Strategy 3/Enable
  Compare To Constant1/1 -> Strategy 2/Enable
  Compare To Constant/1 -> Strategy 1/Enable
  w_set5/1 -> Compare To Constant2/1
  w_set4/1 -> Compare To Constant1/1
  w_set3/1 -> Compare To Constant/1
  Strategy 1/1(frequency) -> Multiport Switch/2
  Multiport Switch/1 -> f/1
  Strategy 1/2(theta) -> Multiport Switch1/2
  Multiport Switch1/1 -> Theta/1
  Strategy 2/2(theta) -> Multiport Switch1/3
  w_set1/1 -> Multiport Switch/1, Multiport Switch1/1
  Strategy 2/1(frequency) -> Multiport Switch/3
  Strategy 3/1(frequency) -> Multiport Switch/4
  Strategy 3/2(theta) -> Multiport Switch1/4
  w_set_pu/1 -> Strategy 3/3(w_set_pu)
  w_PLL/1 -> Strategy 1/4(w_PLL), Strategy 2/3(w_PLL)
  delta_PLL/1 -> Strategy 1/3(delta_PLL)
  P_set/1 -> Strategy 1/2(P_set), Strategy 3/2(P_set), Strategy 2/2(P_set)
  P_mes/1 -> Strategy 1/1(P_mes), Strategy 2/1(P_mes), Strategy 3/1(P_mes)

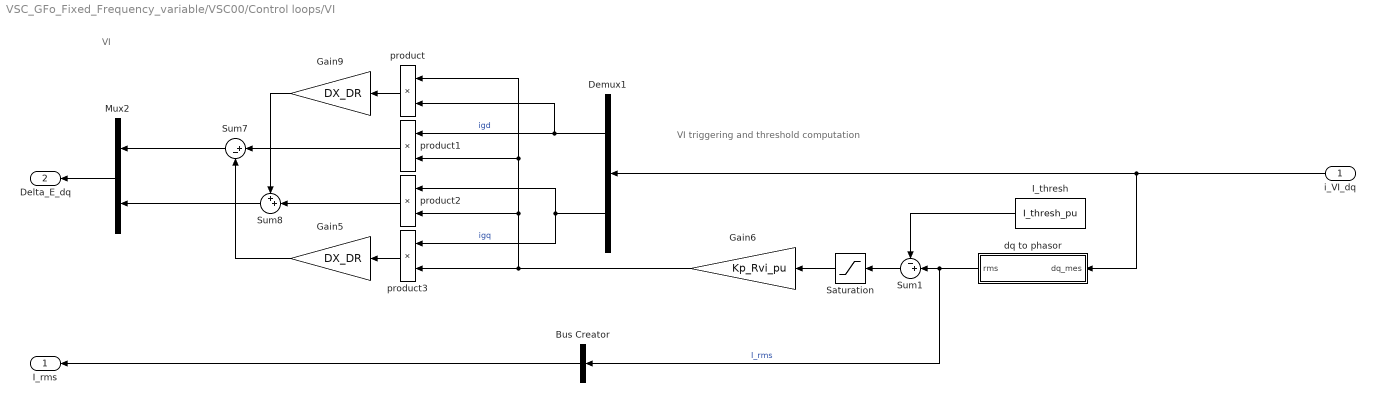
== system VSC_GFo_Fixed_Frequency_variable/VSC00/Control loops/VI ==
  note: VI triggering and threshold computation
  note: VI
  i_VI_dq : Inport
  Bus Creator : BusCreator  Inputs=1
  Demux1 : Demux  Outputs=2
  Gain5 : Gain  Gain=DX_DR
  Gain6 : Gain  Gain=Kp_Rvi_pu
  Gain9 : Gain  Gain=DX_DR
  I_thresh : Constant  Value=I_thresh_pu
  Mux2 : Mux  Inputs=2
  Saturation : Saturate  UpperLimit=inf  LowerLimit=0
  Sum1 : Sum  Inputs=-+|
  Sum7 : Sum  Inputs=|+-
  Sum8 : Sum  Inputs=++|
  dq to phasor : Subsystem
  product{,1..3} (4 alike) : Product  SaturateOnIntegerOverflow=on  RndMeth=Zero  InputSameDT=on  OutDataTypeStr=Inherit: Same as first input
  I_rms : Outport
  Delta_E_dq : Outport  Port=2
  wires:
  Bus Creator/1 -> I_rms/1
  Sum1/1 -> Saturation/1
  dq to phasor/1(rms) -> Sum1/2, Bus Creator/1  "I_rms"
  Saturation/1 -> Gain6/1
  I_thresh/1 -> Sum1/1
  Mux2/1 -> Delta_E_dq/1
  Gain6/1 -> product3/2, product/1, product1/2, product2/2
  product3/1 -> Gain5/1
  product/1 -> Gain9/1
  Demux1/1 -> product1/1, product/2  "igd"
  Demux1/2 -> product2/1, product3/1  "igq"
  product1/1 -> Sum7/1
  Gain5/1 -> Sum7/2
  Gain9/1 -> Sum8/1
  product2/1 -> Sum8/2
  Sum7/1 -> Mux2/1
  Sum8/1 -> Mux2/2
  i_VI_dq/1 -> dq to phasor/1(dq_mes), Demux1/1

== system VSC_GFo_Fixed_Frequency_variable/VSC00/Control loops/abc --> dq (normalized) ==
  abc : Inport
  Theta : Inport  Port=2
  Demux3 : Demux  Outputs=[1 1 1]
  Mux2 : Mux  Inputs=2
  Normalization gain 1 pu rms in abc = 1 pu in dq : Gain  Gain=1/(sqrt(3))
  abc_2_alpha_beta : Subsystem
  alpha_beta_2_dq : Subsystem
  dq : Outport
  wires:
  Normalization gain 1 pu rms in abc = 1 pu in dq/1 -> dq/1
  Theta/1 -> alpha_beta_2_dq/1(Theta)
  Demux3/3 -> abc_2_alpha_beta/3(c)
  abc/1 -> Demux3/1
  alpha_beta_2_dq/2(q) -> Mux2/2
  abc_2_alpha_beta/2(beta) -> alpha_beta_2_dq/3(b)
  alpha_beta_2_dq/1(d) -> Mux2/1
  Demux3/2 -> abc_2_alpha_beta/2(b)
  Demux3/1 -> abc_2_alpha_beta/1(a)
  abc_2_alpha_beta/1(alpha) -> alpha_beta_2_dq/2(a)
  Mux2/1 -> Normalization gain 1 pu rms in abc = 1 pu in dq/1

== system VSC_GFo_Fixed_Frequency_variable/VSC00/Control loops/dq  -->  abc (normalized)  ==
  dq : Inport
  Theta : Inport  Port=2
  Demux2 : Demux  Outputs=[1 1]
  Normalization gain 1 pu in dq = 1 pu rms in abc : Gain  Gain=sqrt(3)
  alpha_beta_2_abc : Subsystem
  dq_2_alpha_beta : Subsystem
  abc : Outport
  wires:
  Normalization gain 1 pu in dq = 1 pu rms in abc/1 -> Demux2/1
  alpha_beta_2_abc/1(abc) -> abc/1
  dq/1 -> Normalization gain 1 pu in dq = 1 pu rms in abc/1
  Theta/1 -> dq_2_alpha_beta/1(Theta)
  Demux2/2 -> dq_2_alpha_beta/3(q)
  Demux2/1 -> dq_2_alpha_beta/2(d)
  dq_2_alpha_beta/2(b) -> alpha_beta_2_abc/2(b)
  dq_2_alpha_beta/1(a) -> alpha_beta_2_abc/1(a)

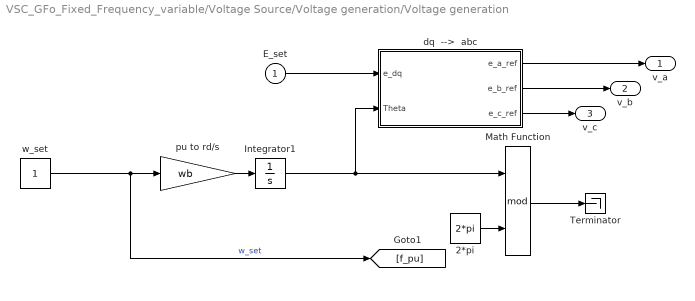
== system VSC_GFo_Fixed_Frequency_variable/Voltage Source/Voltage generation/Voltage generation ==
  E_set : Inport
  " pu to rd/s" : Gain  Gain=wb
  2*pi : Constant  Value=2*pi
  Integrator1 : Integrator
  Math Function : Math  Operator=mod  SaturateOnIntegerOverflow=on
  Terminator : Terminator
  "dq  -->  abc " : Subsystem
  w_set : Constant
  v_a : Outport
  v_b : Outport  Port=2
  v_c : Outport  Port=3
  wires:
  Integrator1/1 -> "dq  -->  abc "/2(Theta), Math Function/1
  " pu to rd/s"/1 -> Integrator1/1
  Math Function/1 -> Terminator/1
  2*pi/1 -> Math Function/2
  "dq  -->  abc "/1(e_a_ref) -> v_a/1
  "dq  -->  abc "/2(e_b_ref) -> v_b/1
  "dq  -->  abc "/3(e_c_ref) -> v_c/1
  w_set/1 -> [f_pu], " pu to rd/s"/1  "w_set"
  E_set/1 -> "dq  -->  abc "/1(e_dq)

== system VSC_GFo_Fixed_Frequency_variable/Voltage Source/Voltage generation/pu --> SI ==
  e_a_pu : Inport
  e_b_pu : Inport  Port=2
  e_c_pu : Inport  Port=3
  nq : Gain  Gain=Vb
  nq1 : Gain  Gain=Vb
  nq2 : Gain  Gain=Vb
  e_a_SI : Outport
  e_b_SI : Outport  Port=2
  e_c_SI : Outport  Port=3
  wires:
  e_b_pu/1 -> nq1/1
  nq2/1 -> e_c_SI/1
  nq/1 -> e_a_SI/1
  e_c_pu/1 -> nq2/1
  nq1/1 -> e_b_SI/1
  e_a_pu/1 -> nq/1

== system VSC_GFo_Fixed_Frequency_variable/VSC00/Control loops/Damping/Filter w_LF ==
  e : Inport
  1/T_LP : Gain  Gain=W_TVR  SaturateOnIntegerOverflow=on  OutDataTypeStr=Inherit: Same as input  ParamDataTypeStr=Inherit: Same as input
  Integrator : Integrator  InitialConditionSource=external  InitialCondition=[VSC01_id0*0.04]
  Sum1 : Sum  Inputs=|+-  SaturateOnIntegerOverflow=on  InputSameDT=on  OutDataTypeStr=Inherit: Same as first input
  s : Outport
  wires:
  e/1 -> Sum1/1, Integrator/2
  Integrator/1 -> s/1, Sum1/2
  1/T_LP/1 -> Integrator/1
  Sum1/1 -> 1/T_LP/1

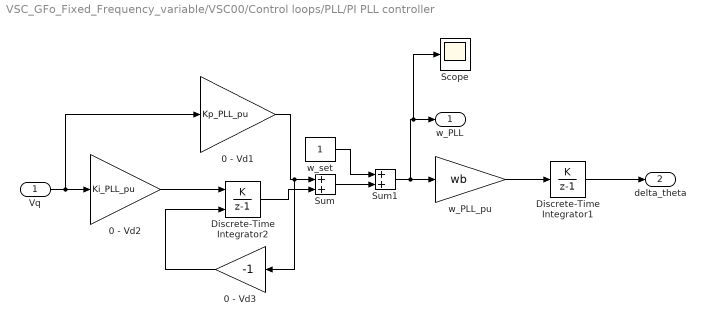
== system VSC_GFo_Fixed_Frequency_variable/VSC00/Control loops/PLL/PI PLL controller ==
  Vq : Inport
  0 - Vd1 : Gain  Gain=Kp_PLL_pu  SaturateOnIntegerOverflow=on  OutDataTypeStr=Inherit: Same as input  ParamDataTypeStr=Inherit: Same as input
  0 - Vd2 : Gain  Gain=Ki_PLL_pu  SaturateOnIntegerOverflow=on  OutDataTypeStr=Inherit: Same as input  ParamDataTypeStr=Inherit: Same as input
  0 - Vd3 : Gain  Gain=-1  SaturateOnIntegerOverflow=on  OutDataTypeStr=Inherit: Same as input  ParamDataTypeStr=Inherit: Same as input
  Discrete-Time Integrator1 : DiscreteIntegrator  IntegratorMethod=Accumulation: Forward Euler  gainval=Time_Step  InitialCondition=Theta0*pi/180  InitialConditionSetting=State (most efficient)  SampleTime=-1  ICPrevOutput=DiscIntNeverNeededParam  ICPrevScaledInput=DiscIntNeverNeededParam
  Discrete-Time Integrator2 : DiscreteIntegrator  IntegratorMethod=Accumulation: Forward Euler  gainval=Time_Step  InitialConditionSource=external  InitialConditionSetting=State (most efficient)  SampleTime=-1  ICPrevOutput=DiscIntNeverNeededParam  ICPrevScaledInput=DiscIntNeverNeededParam
  Scope : Scope
  Sum : Sum  SaturateOnIntegerOverflow=on
  Sum1 : Sum  SaturateOnIntegerOverflow=on
  w_PLL_pu : Gain  Gain=wb  SaturateOnIntegerOverflow=on  OutDataTypeStr=Inherit: Same as input  ParamDataTypeStr=Inherit: Same as input
  w_set : Constant
  w_PLL : Outport
  delta_theta : Outport  Port=2
  wires:
  Sum1/1 -> w_PLL_pu/1, Scope/1, w_PLL/1
  Discrete-Time Integrator1/1 -> delta_theta/1
  Vq/1 -> 0 - Vd1/1, 0 - Vd2/1
  Sum/1 -> Sum1/2
  Discrete-Time Integrator2/1 -> Sum/2
  w_PLL_pu/1 -> Discrete-Time Integrator1/1
  w_set/1 -> Sum1/1
  0 - Vd2/1 -> Discrete-Time Integrator2/1
  0 - Vd1/1 -> 0 - Vd3/1, Sum/1
  0 - Vd3/1 -> Discrete-Time Integrator2/2

== system VSC_GFo_Fixed_Frequency_variable/VSC00/Control loops/PLL/abc --> dq (normalized) ==
  abc : Inport
  Theta : Inport  Port=2
  Demux3 : Demux  Outputs=3
  Mux2 : Mux  Inputs=2
  Normalization gain 1 pu rms in abc = 1 pu in dq : Gain  Gain=1/(sqrt(3))
  abc_2_alpha_beta : Subsystem
  alpha_beta_2_dq : Subsystem
  dq : Outport
  wires:
  Normalization gain 1 pu rms in abc = 1 pu in dq/1 -> dq/1
  Theta/1 -> alpha_beta_2_dq/1(Theta)
  Demux3/3 -> abc_2_alpha_beta/3(c)
  abc/1 -> Demux3/1
  alpha_beta_2_dq/2(q) -> Mux2/2
  abc_2_alpha_beta/2(beta) -> alpha_beta_2_dq/3(b)
  alpha_beta_2_dq/1(d) -> Mux2/1
  Demux3/2 -> abc_2_alpha_beta/2(b)
  Demux3/1 -> abc_2_alpha_beta/1(a)
  abc_2_alpha_beta/1(alpha) -> alpha_beta_2_dq/2(a)
  Mux2/1 -> Normalization gain 1 pu rms in abc = 1 pu in dq/1

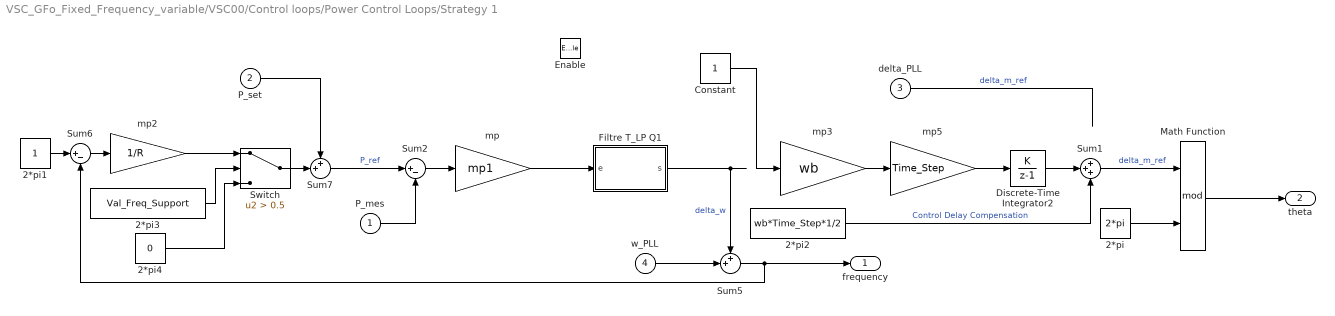
== system VSC_GFo_Fixed_Frequency_variable/VSC00/Control loops/Power Control Loops/Strategy 1 ==
  P_mes : Inport
  P_set : Inport  Port=2
  delta_PLL : Inport  Port=3
  w_PLL : Inport  Port=4
  Enable : EnablePort
  2*pi : Constant  Value=2*pi
  2*pi1 : Constant
  2*pi2 : Constant  Value=wb*Time_Step*1/2
  2*pi3 : Constant  Value=Val_Freq_Support
  2*pi4 : Constant  Value=0
  Constant : Constant
  Discrete-Time Integrator2 : DiscreteIntegrator  IntegratorMethod=Accumulation: Forward Euler  gainval=1  InitialCondition=(Theta_vsc0-Theta0*0)*pi/180  InitialConditionSetting=State (most efficient)  SampleTime=Time_Step  ICPrevOutput=DiscIntNeverNeededParam  ICPrevScaledInput=DiscIntNeverNeededParam
  Filtre T_LP Q1 : Subsystem
  Math Function : Math  Operator=mod  SaturateOnIntegerOverflow=on
  Sum1 : Sum  Inputs=+++
  Sum2 : Sum  Inputs=|+-
  Sum5 : Sum  Inputs=++|
  Sum6 : Sum  Inputs=|+-
  Sum7 : Sum  Inputs=++|
  Switch : Switch  Criteria=u2 > Threshold  Threshold=0.5
  mp : Gain  Gain=mp1
  mp2 : Gain  Gain=1/R
  mp3 : Gain  Gain=wb
  mp5 : Gain  Gain=Time_Step
  frequency : Outport
  theta : Outport  Port=2
  wires:
  2*pi4/1 -> Switch/3
  2*pi3/1 -> Switch/2
  mp2/1 -> Switch/1
  2*pi2/1 -> Sum1/3  "Control Delay Compensation"
  Sum5/1 -> Sum6/2, frequency/1
  w_PLL/1 -> Sum5/2
  delta_PLL/1 -> ?  "delta_m_ref"
  mp/1 -> Filtre T_LP Q1/1(e)
  Filtre T_LP Q1/1(s) -> Sum5/1  "delta_w"
  Math Function/1 -> theta/1
  Switch/1 -> Sum7/2
  P_mes/1 -> Sum2/2
  Sum7/1 -> Sum2/1  "P_ref"
  P_set/1 -> Sum7/1
  Sum6/1 -> mp2/1
  2*pi1/1 -> Sum6/1
  2*pi/1 -> Math Function/2
  Sum1/1 -> Math Function/1  "delta_m_ref"
  Sum2/1 -> mp/1
  mp5/1 -> Discrete-Time Integrator2/1
  Discrete-Time Integrator2/1 -> Sum1/2
  mp3/1 -> mp5/1
  Constant/1 -> mp3/1

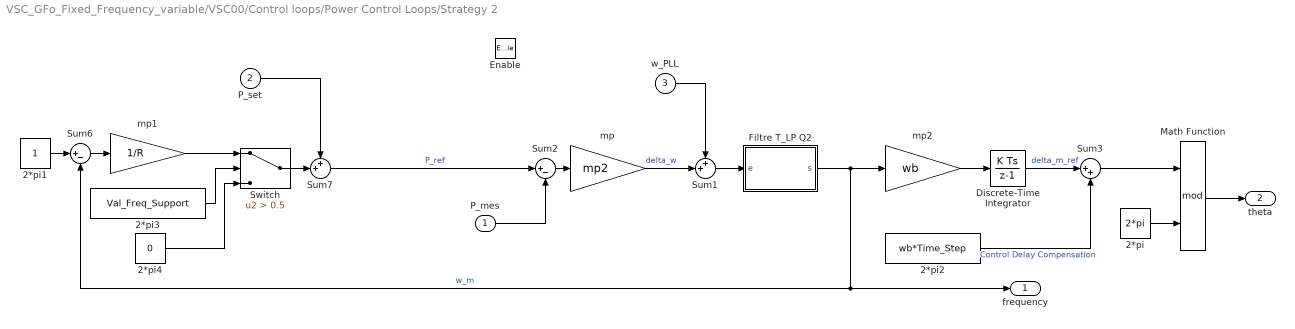
== system VSC_GFo_Fixed_Frequency_variable/VSC00/Control loops/Power Control Loops/Strategy 2 ==
  P_mes : Inport
  P_set : Inport  Port=2
  w_PLL : Inport  Port=3
  Enable : EnablePort
  2*pi : Constant  Value=2*pi
  2*pi1 : Constant
  2*pi2 : Constant  Value=wb*Time_Step
  2*pi3 : Constant  Value=Val_Freq_Support
  2*pi4 : Constant  Value=0
  Discrete-Time Integrator : DiscreteIntegrator  InitialCondition=Theta_vsc0*pi/180  InitialConditionSetting=State (most efficient)  SampleTime=-1  ICPrevOutput=DiscIntNeverNeededParam  ICPrevScaledInput=DiscIntNeverNeededParam
  Filtre T_LP Q2 : Subsystem
  Math Function : Math  Operator=mod  SaturateOnIntegerOverflow=on
  Sum1 : Sum  Inputs=++|
  Sum2 : Sum  Inputs=|+-
  Sum3 : Sum  Inputs=|++
  Sum6 : Sum  Inputs=|+-
  Sum7 : Sum  Inputs=++|
  Switch : Switch  Criteria=u2 > Threshold  Threshold=0.5
  mp : Gain  Gain=mp2
  mp1 : Gain  Gain=1/R
  mp2 : Gain  Gain=wb
  frequency : Outport
  theta : Outport  Port=2
  wires:
  Sum7/1 -> Sum2/1  "P_ref"
  2*pi4/1 -> Switch/3
  2*pi3/1 -> Switch/2
  mp1/1 -> Switch/1
  2*pi1/1 -> Sum6/1
  Sum6/1 -> mp1/1
  P_set/1 -> Sum7/1
  Switch/1 -> Sum7/2
  Sum3/1 -> Math Function/1
  2*pi2/1 -> Sum3/2  "Control Delay Compensation"
  mp2/1 -> Discrete-Time Integrator/1
  P_mes/1 -> Sum2/2
  w_PLL/1 -> Sum1/1
  Filtre T_LP Q2/1(s) -> Sum6/2, frequency/1, mp2/1  "w_m"
  mp/1 -> Sum1/2  "delta_w"
  Sum2/1 -> mp/1
  Discrete-Time Integrator/1 -> Sum3/1  "delta_m_ref"
  Math Function/1 -> theta/1
  2*pi/1 -> Math Function/2
  Sum1/1 -> Filtre T_LP Q2/1(e)

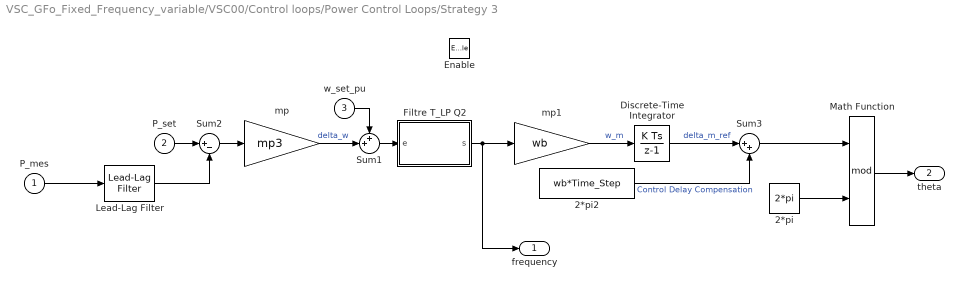
== system VSC_GFo_Fixed_Frequency_variable/VSC00/Control loops/Power Control Loops/Strategy 3 ==
  P_mes : Inport
  P_set : Inport  Port=2
  w_set_pu : Inport  Port=3
  Enable : EnablePort
  2*pi : Constant  Value=2*pi
  2*pi2 : Constant  Value=wb*Time_Step
  Discrete-Time Integrator : DiscreteIntegrator  InitialCondition=Theta_vsc0*pi/180  InitialConditionSetting=State (most efficient)  SampleTime=Time_Step  ICPrevOutput=DiscIntNeverNeededParam  ICPrevScaledInput=DiscIntNeverNeededParam
  Filtre T_LP Q2 : Subsystem
  Lead-Lag Filter : powerlib_meascontrol/Filters/Lead-Lag Filter  T1=T1  T2=T2  Vdc_Init=P0  Ts=0
  Math Function : Math  Operator=mod  SaturateOnIntegerOverflow=on
  Sum1 : Sum  Inputs=++|
  Sum2 : Sum  Inputs=|+-
  Sum3 : Sum  Inputs=|++
  mp : Gain  Gain=mp3
  mp1 : Gain  Gain=wb
  frequency : Outport
  theta : Outport  Port=2
  wires:
  Lead-Lag Filter/1 -> Sum2/2
  2*pi2/1 -> Sum3/2  "Control Delay Compensation"
  Sum3/1 -> Math Function/1
  mp1/1 -> Discrete-Time Integrator/1  "w_m"
  Sum1/1 -> Filtre T_LP Q2/1(e)
  P_mes/1 -> Lead-Lag Filter/1
  Filtre T_LP Q2/1(s) -> mp1/1, frequency/1
  mp/1 -> Sum1/2  "delta_w"
  P_set/1 -> Sum2/1
  w_set_pu/1 -> Sum1/1
  2*pi/1 -> Math Function/2
  Math Function/1 -> theta/1
  Discrete-Time Integrator/1 -> Sum3/1  "delta_m_ref"
  Sum2/1 -> mp/1

== system VSC_GFo_Fixed_Frequency_variable/VSC00/Control loops/VI/dq to phasor ==
  dq_mes : Inport
  Demux : Demux  Outputs=2
  Sqrt : Sqrt  SaturateOnIntegerOverflow=on
  Sum4 : Sum  Inputs=|++  SaturateOnIntegerOverflow=on  InputSameDT=on  OutDataTypeStr=Inherit: Same as first input
  Vrdird : Product  SaturateOnIntegerOverflow=on  RndMeth=Zero  InputSameDT=on  OutDataTypeStr=Inherit: Same as first input
  Vrqirq : Product  SaturateOnIntegerOverflow=on  RndMeth=Zero  InputSameDT=on  OutDataTypeStr=Inherit: Same as first input
  rms : Outport
  wires:
  Sum4/1 -> Sqrt/1
  Vrqirq/1 -> Sum4/2
  Vrdird/1 -> Sum4/1
  Demux/2 -> Vrqirq/2, Vrqirq/1
  Demux/1 -> Vrdird/2, Vrdird/1
  dq_mes/1 -> Demux/1
  Sqrt/1 -> rms/1

== system VSC_GFo_Fixed_Frequency_variable/VSC00/Control loops/abc --> dq (normalized)/abc_2_alpha_beta ==
  a : Inport
  b : Inport  Port=2
  c : Inport  Port=3
  Fcn1 : Fcn  Expr=sqrt(2/3)*(u(1)+u(2)+u(3))
  Fcn3 : Fcn  Expr=sqrt(2/3)*(u(1)-u(2)/2-u(3)/2)
  Fcn5 : Fcn  Expr=(u(2)-u(3))/sqrt(2)
  Mux : Mux  Inputs=3
  Scope5 : Scope
  alpha : Outport
  beta : Outport  Port=2
  wires:
  Fcn5/1 -> beta/1
  Fcn3/1 -> alpha/1
  b/1 -> Mux/2
  a/1 -> Mux/1
  Mux/1 -> Fcn5/1, Fcn3/1, Fcn1/1
  Fcn1/1 -> Scope5/1
  c/1 -> Mux/3

== system VSC_GFo_Fixed_Frequency_variable/VSC00/Control loops/abc --> dq (normalized)/alpha_beta_2_dq ==
  Theta : Inport
  a : Inport  Port=2
  b : Inport  Port=3
  Fcn1 : Fcn  Expr=u(2)*cos(u(1))+u(3)*sin(u(1))
  Fcn3 : Fcn  Expr=u(2)*sin(u(1))-u(3)*cos(u(1))
  Mux : Mux  Inputs=[1 1 1]
  d : Outport
  q : Outport  Port=2
  wires:
  Fcn1/1 -> q/1
  Fcn3/1 -> d/1
  b/1 -> Mux/3
  a/1 -> Mux/2
  Mux/1 -> Fcn1/1, Fcn3/1
  Theta/1 -> Mux/1

== system VSC_GFo_Fixed_Frequency_variable/VSC00/Control loops/dq  -->  abc (normalized) /alpha_beta_2_abc ==
  a : Inport
  b : Inport  Port=2
  Fcn1 : Fcn  Expr=(-u(1)-sqrt(3)*u(2))/2
  Fcn3 : Fcn  Expr=u(1)
  Fcn5 : Fcn  Expr=(-u(1)+sqrt(3)*u(2))/2
  Gain1 : Gain  Gain=sqrt(2/3)
  Gain2 : Gain  Gain=sqrt(2/3)
  Gain3 : Gain  Gain=sqrt(2/3)
  Mux : Mux  Inputs=2
  Mux1 : Mux  Inputs=[1 1 1]
  abc : Outport
  wires:
  Mux1/1 -> abc/1
  Gain3/1 -> Mux1/1
  Gain2/1 -> Mux1/2
  Gain1/1 -> Mux1/3
  Fcn1/1 -> Gain1/1
  Fcn5/1 -> Gain2/1
  Fcn3/1 -> Gain3/1
  b/1 -> Mux/2
  a/1 -> Mux/1
  Mux/1 -> Fcn1/1, Fcn5/1, Fcn3/1

== system VSC_GFo_Fixed_Frequency_variable/VSC00/Control loops/dq  -->  abc (normalized) /dq_2_alpha_beta ==
  Theta : Inport
  d : Inport  Port=2
  q : Inport  Port=3
  Fcn1 : Fcn  Expr=-u(2)*cos(u(1))+u(3)*sin(u(1))
  Fcn3 : Fcn  Expr=u(2)*sin(u(1))+u(3)*cos(u(1))
  Mux : Mux  Inputs=[1 1 1]
  a : Outport
  b : Outport  Port=2
  wires:
  Mux/1 -> Fcn1/1, Fcn3/1
  Theta/1 -> Mux/1
  d/1 -> Mux/2
  q/1 -> Mux/3
  Fcn3/1 -> a/1
  Fcn1/1 -> b/1

== system VSC_GFo_Fixed_Frequency_variable/Voltage Source/Voltage generation/Voltage generation/dq  -->  abc  ==
  e_dq : Inport
  Theta : Inport  Port=2
  Demux2 : Demux  Outputs=2
  Scope1 : Scope
  abc_alpha_beta : Subsystem
  abc_dq2 : Subsystem
  e_a_ref : Outport
  e_b_ref : Outport  Port=2
  e_c_ref : Outport  Port=3
  wires:
  abc_dq2/1(a) -> abc_alpha_beta/1(a)
  abc_dq2/2(b) -> abc_alpha_beta/2(b)
  Demux2/1 -> abc_dq2/2(d)
  Demux2/2 -> abc_dq2/3(q)
  Theta/1 -> abc_dq2/1(Theta)
  abc_alpha_beta/2(b1) -> e_b_ref/1
  e_dq/1 -> Demux2/1, Scope1/1
  abc_alpha_beta/3(c) -> e_c_ref/1
  abc_alpha_beta/1(a1) -> e_a_ref/1

== system VSC_GFo_Fixed_Frequency_variable/VSC00/Control loops/PLL/abc --> dq (normalized)/abc_2_alpha_beta ==
  a : Inport
  b : Inport  Port=2
  c : Inport  Port=3
  Fcn1 : Fcn  Expr=sqrt(2/3)*(u(1)+u(2)+u(3))
  Fcn3 : Fcn  Expr=sqrt(2/3)*(u(1)-u(2)/2-u(3)/2)
  Fcn5 : Fcn  Expr=(u(2)-u(3))/sqrt(2)
  Mux : Mux  Inputs=3
  Scope5 : Scope
  alpha : Outport
  beta : Outport  Port=2
  wires:
  Fcn5/1 -> beta/1
  Fcn3/1 -> alpha/1
  b/1 -> Mux/2
  a/1 -> Mux/1
  Mux/1 -> Fcn5/1, Fcn3/1, Fcn1/1
  Fcn1/1 -> Scope5/1
  c/1 -> Mux/3

== system VSC_GFo_Fixed_Frequency_variable/VSC00/Control loops/PLL/abc --> dq (normalized)/alpha_beta_2_dq ==
  Theta : Inport
  a : Inport  Port=2
  b : Inport  Port=3
  Fcn1 : Fcn  Expr=u(2)*cos(u(1))+u(3)*sin(u(1))
  Fcn3 : Fcn  Expr=u(2)*sin(u(1))-u(3)*cos(u(1))
  Mux : Mux  Inputs=3
  d : Outport
  q : Outport  Port=2
  wires:
  Fcn1/1 -> q/1
  Fcn3/1 -> d/1
  b/1 -> Mux/3
  a/1 -> Mux/2
  Mux/1 -> Fcn1/1, Fcn3/1
  Theta/1 -> Mux/1
